simulink model "Webcam_motor_test"  (Simulink 7.3)
settings: Solver=FixedStepDiscrete  StartTime=0.0  StopTime=inf  MaxStep=0.2  RelTol=1e-3
settings Model: Creator=gclayton  LastModifiedBy=wildcat
settings DebuggingCC: InheritedTsInSrcMsg=none
settings RTWCC: SystemTargetFile=rlnx.tlc  GenCodeOnly=on  TemplateMakefile=rlnx_ubuntu.tmf  Description=Linux Real-Time Target  ProcessScript=rlnx_make_rtw_hook
settings RTWCC: CustomInclude=|
  | /usr/local/include/opencv/
  | /usr/local/include/
settings CodeAppCC: GenerateComments=off  SimulinkBlockComments=off
settings STFCustomTargetCC: ModelReferenceCompliant=off  MatFileLogging=on  SystemTargetFile=rlnx.tlc
settings GRTTargetCC: ModelReferenceCompliant=off  ParMdlRefBuildCompliant=off  CompOptLevelCompliant=off
settings CustomProperty: DataType=string  Value=-lm -ldl /usr/local/lib/libopencv_highgui.so.2.4
settings EnumStrPairs: String=PC

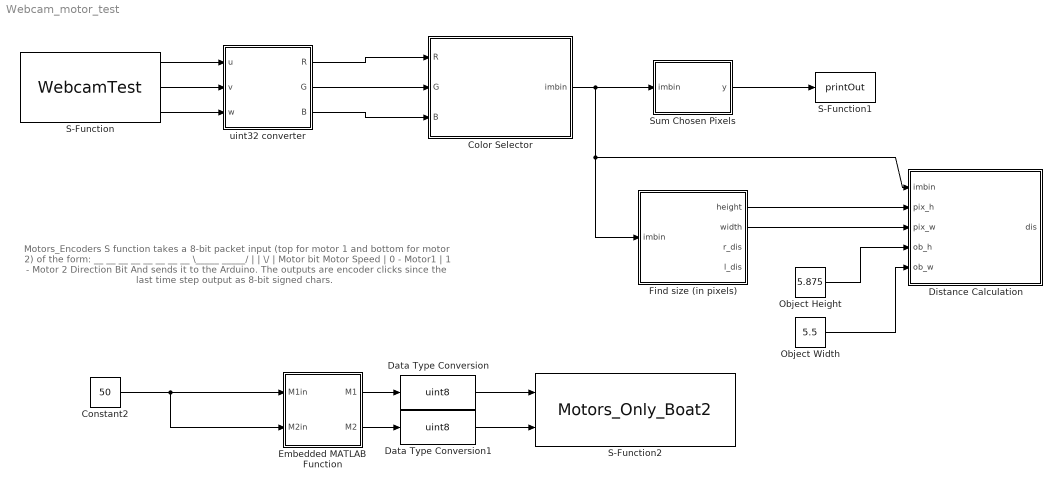
== system Webcam_motor_test ==
  note: Motors_Encoders S function takes a 8-bit packet input
      | (top for motor 1 and bottom for motor 2) of the form:
      |
      |          __ __ __ __ __ __ __ __
      |         \_____   _____/   |    |
      |                               \/              |  Motor bit
      |                          Motor Speed    |   0 - Motor1
      |                                                    |   1 - Motor 2
      |                                Direction Bit
      |
      | And sends it to the Arduino.  The outputs are encoder clicks
      | since the last time step output as 8-bit signed chars.
  Color Selector : Stateflow chart  TreatAsAtomicUnit=on
  Constant2 : Constant  Value=50  OutDataType=fixdt(1, 16)  OutScaling=2^0
  Data Type Conversion : DataTypeConversion  OutDataTypeMode=uint8  OutDataType=fixdt(1, 16)  OutScaling=2^0  OutDataTypeStr=uint8
  Data Type Conversion1 : DataTypeConversion  OutDataTypeMode=uint8  OutDataType=fixdt(1, 16)  OutScaling=2^0  OutDataTypeStr=uint8
  Distance Calculation : Stateflow chart  TreatAsAtomicUnit=on
  Embedded MATLAB Function : Stateflow chart
  Find size (in pixels) : Stateflow chart  TreatAsAtomicUnit=on
  Object Height : Constant  Value=5.875  OutDataType=fixdt(1, 16)  OutScaling=2^0
  Object Width : Constant  Value=5.5  OutDataType=fixdt(1, 16)  OutScaling=2^0
  S-Function : S-Function  FunctionName=WebcamTest  EnableBusSupport=off
  S-Function1 : S-Function  FunctionName=printOut  EnableBusSupport=off
  S-Function2 : S-Function  FunctionName=Motors_Only_Boat2  EnableBusSupport=off
  Sum Chosen Pixels : Stateflow chart
  uint32 converter : Stateflow chart
  wires:
  S-Function/1 -> uint32 converter/1(u)
  S-Function/2 -> uint32 converter/2(v)
  S-Function/3 -> uint32 converter/3(w)
  uint32 converter/2(G) -> Color Selector/2(G)
  uint32 converter/3(B) -> Color Selector/3(B)
  Color Selector/1(imbin) -> Sum Chosen Pixels/1(imbin), Find size (in pixels)/1(imbin), Distance Calculation/1(imbin)
  uint32 converter/1(R) -> Color Selector/1(R)
  Sum Chosen Pixels/1(y) -> S-Function1/1
  Embedded MATLAB Function/1(M1) -> Data Type Conversion/1
  Embedded MATLAB Function/2(M2) -> Data Type Conversion1/1
  Constant2/1 -> Embedded MATLAB Function/1(M1in), Embedded MATLAB Function/2(M2in)
  Data Type Conversion/1 -> S-Function2/1
  Data Type Conversion1/1 -> S-Function2/2
  Find size (in pixels)/1(height) -> Distance Calculation/2(pix_h)
  Find size (in pixels)/2(width) -> Distance Calculation/3(pix_w)
  Object Height/1 -> Distance Calculation/4(ob_h)
  Object Width/1 -> Distance Calculation/5(ob_w)

== matlab function uint32 converter ==
  data: u input double; R output double; v input double; w input double; G output double; B output double
function [R,G,B]= fcn(u,v,w)

R = uint32(u);
G = uint32(v);
B = uint32(w);

== matlab function Sum Chosen Pixels ==
  data: imbin input double; y output double
function y = fcn(imbin)
%#eml

imsize = size(imbin);
red_pix = 0;

for (imh = 1:imsize(1,1));
    for (iml = 1:imsize(1,2));
        im_pix = imbin(imh,iml);     
        if (im_pix == 1)
           red_pix = red_pix+1;
        end
    end
end

y = uint32(red_pix);

== matlab function Color Selector ==
  data: R input double; G input double; B input double; imbin output double
function imbin  = color_selection(R,G,B)

imsize = size(R);
imsize = size(G);
imsize = size(B);

R1 = zeros(imsize);
G1 = zeros(imsize);
B1 = zeros(imsize);
imbin = zeros(imsize);

for (imh = 1:imsize(1,1));
    for (iml = 1:imsize(1,2));
        imR = R(imh,iml);
        imG = G(imh,iml);
        imB = B(imh,iml);
        if (imR >= 170) && (imR <= 255) && (imG >= 15) && (imG <= 70) && (imB >= 70) && (imB <= 130)
            R1(imh,iml) = 255;
            G1(imh,iml) = 255;
            B1(imh,iml) = 255;
            imbin(imh,iml) = 1;
        end
    end
end

== matlab function Find size (in pixels) ==
  data: imbin input double; height output double; width output double; r_dis output double; l_dis output double
function [height,width,r_dis,l_dis] = hw_find(imbin)

imsize=size(imbin);

height = 0;
width = 0;
height_sum = 0;
width_sum = 0;
marker = 0;
obstart = 0;

for (imh = 1:imsize(1,1));
    width_sum = 0;
    for (iml = 1:imsize(1,2));
        imloc = imbin(imh,iml);
        if (imloc == 1)
            width_sum=width_sum+1;
        end
    end
    if (width_sum >= 6)
        height = height+1;
    end
end



for (iml = 1:imsize(1,2));
    height_sum = 0;
    for (imh = 1:imsize(1,1));
        imloc = imbin(imh,iml);
        if (imloc == 1)
            height_sum=height_sum+1;
        end
    end
    if (height_sum >= 6)
        width = width+1;
        if (marker == 0)
            marker = 1;
            obstart = iml;
        end
    end
end

obend = obstart + width;

r_dis = obstart;
l_dis = imsize(1,2) - obend;

== matlab function Embedded MATLAB Function ==
  data: M1in input double; M1 output double; M2in input double; M2 output double
function [M1, M2] = MotorPackets(M1in, M2in)
%#eml

M1 = 0;
M2 = 1;

if M1in <= 0
    M1 = M1+2;
end

if M2in <= 0
    M2 = M2+2;
end

M1 = M1 + round(abs(M1in)*0.1047)*4;
M2 = M2 + round(abs(M2in)*0.1047)*4;

== matlab function Distance Calculation ==
  data: imbin input double; pix_h input double; dis output double; pix_w input double; ob_h input double; ob_w input double
function dis  = find_dis(imbin,pix_h,pix_w,ob_h,ob_w)

%1.4=2*tan(44.443*pi/360)*dis*height1/480;
%ob_w=2*tan(57.154*pi/360)*dis*width1/640;

imsize = size(imbin);

dis1 = (ob_h*imsize(1,1))/(2*tan(44.443*pi/360)*pix_h);

dis2 = (ob_w*imsize(1,2))/(2*tan(57.154*pi/360)*pix_w);

dis=(dis1+dis2)/2;
